simulink subsystem "Pendulum"  (R2023a)
settings: Solver=VariableStepAuto  StartTime=0.0  StopTime=10.0  RelTol=1e-3
values from neighbouring files (symbols this model uses):
  BETA = 0.3    [DemoPendulumSimulink.m]
settings Model: Creator=KozlovM  LastModifiedBy=maxim

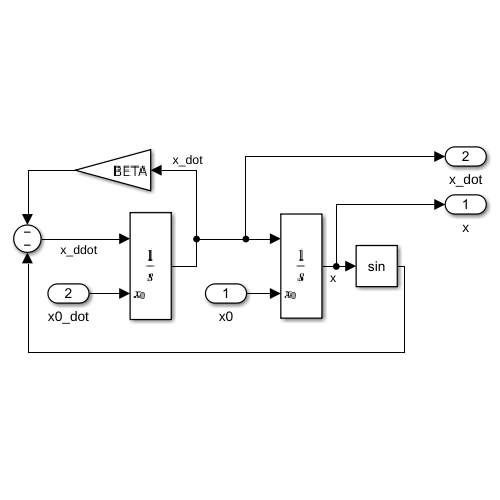
[thumbnail: Simulink's stored preview of the top-level diagram]
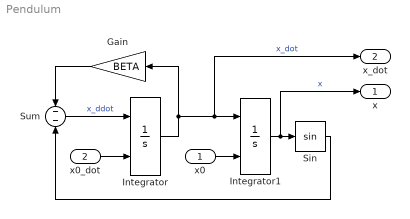
== system Pendulum ==
  x0 : Inport
  x0_dot : Inport  Port=2
  Gain : Gain  Gain=BETA
  Integrator : Integrator  InitialConditionSource=external
  Integrator1 : Integrator  InitialConditionSource=external
  Sin : Trigonometry
  Sum : Sum  Inputs=--
  x : Outport
  x_dot : Outport  Port=2
  wires:
  Integrator1/1 -> Sin/1, x/1  "x"
  Integrator/1 -> Integrator1/1, x_dot/1, Gain/1  "x_dot"
  x0_dot/1 -> Integrator/2
  Gain/1 -> Sum/1
  Sin/1 -> Sum/2
  x0/1 -> Integrator1/2
  Sum/1 -> Integrator/1  "x_ddot"
